simulink model "parameter_estimation"  (R2023b)
settings: Solver=FixedStepAuto  StartTime=0.0  StopTime=66  FixedStep=0.01  RelTol=1e-3
values from neighbouring files (symbols this model uses):
  motor_B = 0.0001    [example_data_LAB1.mat]    (also in motor_params.m)
  motor_J = 0.001    [example_data_LAB1.mat]    (also in motor_params.m)
  motor_K = 0.05    [example_data_LAB1.mat]    (also in motor_params.m)
  motor_L = 0.016    [example_data_LAB1.mat]    (also in motor_params.m)
  motor_R = 22    [example_data_LAB1.mat]    (also in motor_params.m)
undefined symbols (not defined in the file or in its folder): DiscIntNeverNeededParam
libraries: simulink x1
settings Model: Creator=tanawatp  LastModifiedBy=tanawatp

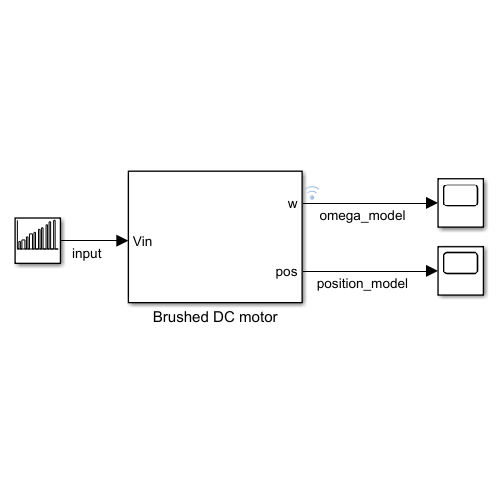
[thumbnail: Simulink's stored preview of the top-level diagram]
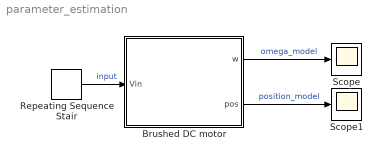
== system parameter_estimation ==
  Brushed DC motor : Subsystem
  Repeating Sequence Stair : simulink/Sources/Repeating Sequence Stair  OutValues=[0 3 0 4 0 5 0 6 0 7 0 8 0 9 0 10 0 11 0 12 0 0]  tsamp=3  OutMin=[]  OutMax=[]  OutDataTypeStr=double  OutputDataTypeScalingMode=double  OutDataType=fixdt(0,8)  ConRadixGroup=Best Precision: Vector-wise  OutScaling=2^-12
  Scope : Scope
  Scope1 : Scope
  wires:
  Brushed DC motor/1(w) -> Scope/1  "omega_model"
  Brushed DC motor/2(pos) -> Scope1/1  "position_model"
  Repeating Sequence Stair/1 -> Brushed DC motor/1(Vin)  "input"

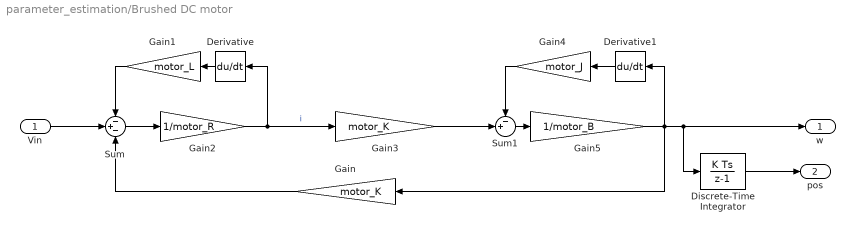
== system parameter_estimation/Brushed DC motor ==
  Vin : Inport
  Derivative : Derivative
  Derivative1 : Derivative
  Discrete-Time Integrator : DiscreteIntegrator  SampleTime=-1  ICPrevOutput=DiscIntNeverNeededParam  ICPrevScaledInput=DiscIntNeverNeededParam
  Gain : Gain  Gain=motor_K
  Gain1 : Gain  Gain=motor_L
  Gain2 : Gain  Gain=1/motor_R
  Gain3 : Gain  Gain=motor_K
  Gain4 : Gain  Gain=motor_J
  Gain5 : Gain  Gain=1/motor_B
  Sum : Sum  Inputs=-+-
  Sum1 : Sum  Inputs=-+|
  w : Outport
  pos : Outport  Port=2
  wires:
  Derivative/1 -> Gain1/1
  Gain5/1 -> w/1, Discrete-Time Integrator/1, Gain/1, Derivative1/1
  Gain1/1 -> Sum/1
  Gain4/1 -> Sum1/1
  Sum/1 -> Gain2/1
  Gain3/1 -> Sum1/2
  Sum1/1 -> Gain5/1
  Discrete-Time Integrator/1 -> pos/1
  Gain/1 -> Sum/3
  Derivative1/1 -> Gain4/1
  Gain2/1 -> Derivative/1, Gain3/1  "i"
  Vin/1 -> Sum/2
